simulink model "helicoptertemplate_mpc"  (R2021b)
settings: Solver=ode45  StartTime=0.0  StopTime=Tsim  RelTol=1e-3
InitFcn:
  | hwinit
values from neighbouring files (symbols this model uses):
  A = sysd.A    [MPC_Reference_track.m]    (also in MPC_Reference_track_offset.m; MPC_init_v2.m; MPC_init_v3.m; modelDynamics.m = [0, 1; -(1/J)*g*Mcw*L1*cos(-0.38), -(1/J)*C_alpha])
  B = sysd.B    [MPC_Reference_track.m]    (also in MPC_Reference_track_offset.m; MPC_init_v2.m; MPC_init_v3.m; modelDynamics.m = [0; (1/J)*L2])
  C = sysd.C    [MPC_Reference_track.m]    (also in MPC_Reference_track_offset.m; MPC_init_v2.m; MPC_init_v3.m; modelDynamics.m = [1, 0])
  H = predmod.S'*Qbar*predmod.S+Rbar    [costgen.m]    (also in costgen_delta.m = S' * Qbar * S + Delta' * Rbar * Delta)
  h = 0.01    [MPC_Reference_track.m]    (also in MPC_Reference_track_offset.m; MPC_init_v2.m; MPC_init_v3.m; costgen.m = [hx0 hxref huref])
  sysd = c2d(sys, h)    [MPC_Reference_track.m]    (also in MPC_Reference_track_offset.m; MPC_init_v2.m; MPC_init_v3.m)
undefined symbols (not defined in the file or in its folder): adingain, adinoffs, DiscIntNeverNeededParam, Discrete, h_cost, HeliMexHandle, Time
libraries: ctrlSharedLib x1
settings Model: Creator=fkzhang  LastModifiedBy=rjvanderhorst
settings SolverCC: AlgebraicLoopSolver=TrustRegion
settings DataIOCC: LimitDataPoints=on  SaveFormat=Array  ReturnWorkspaceOutputs=off
settings OptimizationCC: BlockReduction=off  BooleanDataType=off  LifeSpan=inf
settings DebuggingCC: SaveWithParameterizedLinksMsg=none  UnderspecifiedInitializationDetection=Classic  MergeDetectMultiDrivingBlocksExec=none  SignalResolutionControl=TryResolveAllWithWarning  AllowSymbolicDim=off  SFUnexpectedBacktrackingDiag=warning  SFNoUnconditionalDefaultTransitionDiag=warning  SFExecutionAtInitializationDiag=none  SFMachineParentedDataDiag=warning  ArithmeticOperatorsInVariantConditions=warning
settings HardwareCC: ProdBitPerPointer=32  ProdBitPerSizeT=32  ProdBitPerPtrDiffT=32  ProdLargestAtomicFloat=None  ProdIntDivRoundTo=Undefined  ProdEndianess=Unspecified  ProdWordSize=32  ProdHWDeviceType=32-bit Generic  TargetUnknown=on
settings ModelReferenceCC: PropagateSignalLabelsOutOfModel=off
settings SFSimCC: SimUseLocalCustomCode=off  CustomCodeUndefinedFunction=UseInterfaceOnly
settings RTWCC: RTWUseLocalCustomCode=off
settings CodeAppCC: StateflowObjectComments=on
settings GRTTargetCC: TargetLangStandard=C89/C90 (ANSI)
settings ConfigComp: CovMetricSettings=dw  CovSaveCumulativeToWorkspaceVar=on  CovSaveSingleToWorkspaceVar=on  CovExternalEMLEnable=off  CovSFcnEnable=off

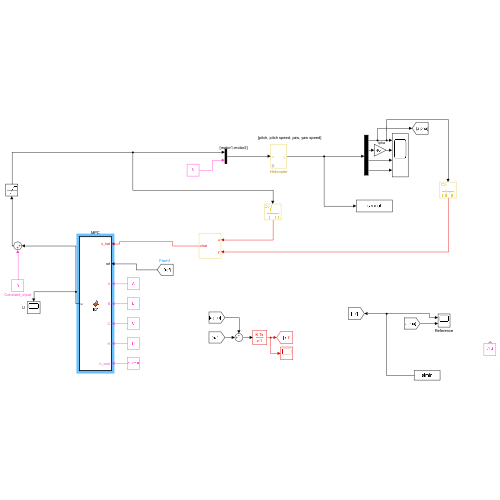
[thumbnail: Simulink's stored preview of the top-level diagram]
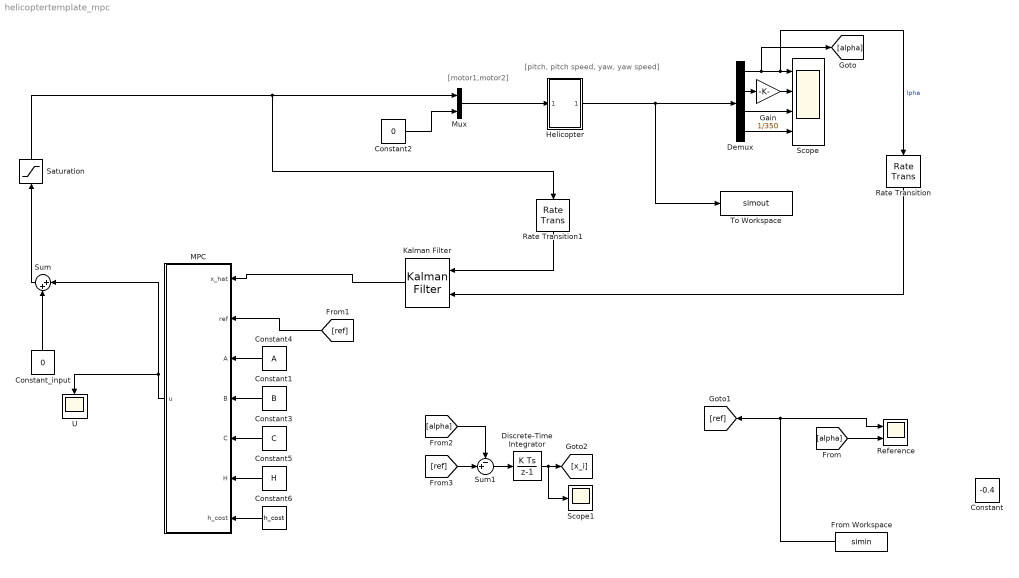
== system helicoptertemplate_mpc ==
  note: [pitch, pitch speed, yaw, yaw speed]
  note: [motor1,motor2]
  Constant : Constant  Value=-0.4
  Constant1 : Constant  Value=B  VectorParams1D=off
  Constant2 : Constant  Value=0
  Constant3 : Constant  Value=C  VectorParams1D=off
  Constant4 : Constant  Value=A
  Constant5 : Constant  Value=H
  Constant6 : Constant  Value=h_cost
  Constant_input : Constant  Value=0
  Demux : Demux
  Discrete-Time Integrator : DiscreteIntegrator  SampleTime=-1  ICPrevOutput=DiscIntNeverNeededParam  ICPrevScaledInput=DiscIntNeverNeededParam
  From Workspace : FromWorkspace  VariableName=simin
  Gain : Gain  Gain=1/350
  Helicopter : Subsystem  mask{Ts=h}
      mask prompts: Ts "sampletime"
      mask init:
      | sf_heli_init
      mask Display:
      | port_label('input',1,'u');
      | port_label('output',1,'y');
  Kalman Filter : ctrlSharedLib/Kalman Filter  TimeDomain=Discrete-Time  UseCurrentEstimator=on  ModelSource=Individual A, B, C, D matrices  ModelSourceVariable=ss(0.95,1,1,0,1)  A=sysd.A  B=sysd.B  C=sysd.C  D=sysd.D  NumberOfStates=1  NumberOfInputs=1  NumberOfOutputs=1  InitialEstimateSource=Dialog  X0=[0; 0]  P0=10  UseK=off  UseGH=off  NumberOfProcessNoiseInputs=1  G=1  TimeInvariantG=on  H=0  TimeInvariantH=on  Q=0.05  TimeInvariantQ=on  R=1  TimeInvariantR=on  N=0  TimeInvariantN=on  AddInputPort=on  AddEnablePort=off  OutputEstimatedY=off  OutputP=off  Ts=h
  MPC : MATLAB Function  TreatAsAtomicUnit=on
  Mux : Mux  Inputs=2
  Rate Transition : RateTransition  OutPortSampleTime=h
  Rate Transition1 : RateTransition  OutPortSampleTime=h
  Reference : Scope  NumInputPorts=2
  Saturation : Saturate  UpperLimit=1  LowerLimit=-1
  Scope : Scope  NumInputPorts=4
  Scope1 : Scope
  Sum : Sum  Inputs=|++
  Sum1 : Sum  Inputs=-+|
  To Workspace : ToWorkspace  VariableName=simout  SaveFormat=Structure With Time  SampleTime=-1
  U : Scope
  wires:
  Helicopter/1(Out1) -> To Workspace/1, Demux/1
  Mux/1 -> Helicopter/1(In1)
  Constant2/1 -> Mux/2
  Demux/3 -> Scope/3
  Demux/4 -> Scope/4
  Demux/2 -> Gain/1
  Gain/1 -> Scope/2
  Demux/1 -> [alpha], Rate Transition/1, Scope/1  "lpha"
  Constant_input/1 -> Sum/2
  Sum/1 -> Saturation/1
  MPC/1(u) -> Sum/1, U/1
  Kalman Filter/1 -> MPC/1(x_hat)
  Saturation/1 -> Rate Transition1/1, Mux/1
  Rate Transition/1 -> Kalman Filter/2
  [alpha] -> Reference/2
  From Workspace/1 -> Reference/1, [ref]
  [alpha] -> Sum1/1
  [ref] -> Sum1/2
  Sum1/1 -> Discrete-Time Integrator/1
  Discrete-Time Integrator/1 -> Scope1/1, [x_i]
  Constant1/1 -> MPC/4(B)
  Constant3/1 -> MPC/5(C)
  Constant4/1 -> MPC/3(A)
  Constant5/1 -> MPC/6(H)
  Constant6/1 -> MPC/7(h_cost)
  Rate Transition1/1 -> Kalman Filter/1
  [ref] -> MPC/2(ref)

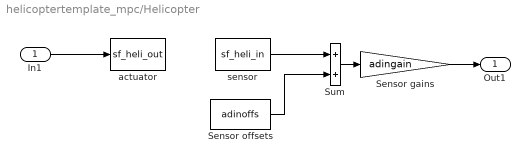
== system helicoptertemplate_mpc/Helicopter ==
  In1 : Inport
  Sensor gains : Gain  Gain=adingain
  Sensor offsets : Constant  Value=adinoffs
  Sum : Sum
  actuator : M-S-Function  FunctionName=sf_heli_out  Parameters=HeliMexHandle,Ts
  sensor : M-S-Function  FunctionName=sf_heli_in  Parameters=HeliMexHandle
  Out1 : Outport
  wires:
  sensor/1 -> Sum/1
  In1/1 -> actuator/1
  Sensor offsets/1 -> Sum/2
  Sum/1 -> Sensor gains/1
  Sensor gains/1 -> Out1/1

== matlab function helicoptertemplate_mpc/MPC ==
  data: x_hat input; ref input; A input; B input; u output; C input; H input; h_cost input
function u = fcn(x_hat, ref, A, B, C, H, h_cost)
      
    u = zeros(1,1); % Define the output type for the extrinsic call.
    
    N = 20; %prediction horizon
    coder.extrinsic('quadprog');
    A_OT = [eye(2)-A, -B; C, zeros(1,1)];
    disp(size(A_OT))
    B_OT = [zeros(2,1); ref];
    
    H_ots = [0 0 0;
             0 0 0;
             0 0 1];
    
    lb_ots = [-10000; 0; -1];
    ub_ots = -lb_ots;
    
    %options = optimoptions('fmincon', 'Algorithm','sqp');
    OTS = quadprog(H_ots,[],[],[],A_OT,B_OT,lb_ots,ub_ots,[]);
    x_ref = OTS(1:2);
    u_ref = OTS(3);
    %%%%%%%%%%%%%%%%%%%%%%%%%%%OTS%%%%%%%%%%%%%%%%%%%%%%%%%%%%


    

    %%%%%%%%%%%%%%%%%%%%%%%%%%%MPC%%%%%%%%%%%%%%%%%%%%%%%%%%%%
    x_0=x_hat;
    
    lb = -1*ones(N,1);
    ub = -0*lb;
    uN = quadprog(H,(h_cost*[x_0; x_ref; u_ref]),[],[],[],[],lb,ub,[]);

    % Select the first input only
    u=uN(1);

end
